simulink model "DisplayModel_Step4_start"  (R2013b)
settings: Solver=FixedStepDiscrete  StartTime=0.0  StopTime=10.0  FixedStep=0.2  RelTol=1e-3
settings Model: CovPath=LandingGearModes  CovMetricSettings=dcmw  CovHTMLOptions=-sRT=1 -aTS=1 -bRG=1 -bTC=1 -hTR=0 -nFC=0 -scm=1 -bcm=1 -xEv=0  CovModelRefEnable=off  Creator=siddhars  LastModifiedBy=rruff
settings OptimizationCC: InlineParams=on  ExpressionDepthLimit=2147483647  OptimizeModelRefInitCode=on  LifeSpan=1
settings DebuggingCC: StateNameClashWarn=warning
settings RTWCC: SystemTargetFile=ert.tlc  TemplateMakefile=ert_default_tmf  Description=Embedded Coder  ProcessScript=ert_make_rtw_hook  PortableWordSizes=on
settings CodeAppCC: IgnoreCustomStorageClasses=off  CustomSymbolStrType=$N$R$M  InternalIdentifier=Classic
settings ERTTargetCC: CodeReplacementLibrary=ANSI_C  GenerateSampleERTMain=on  InlinedParameterPlacement=NonHierarchical  ERTCustomFileTemplate=example_file_process.tlc
settings ConfigComp: Description=Design Verifier Custom Configuration Component  DVModelCoverageObjectives=MCDC  DVMaxTestCaseSteps=500  DVTestSuiteOptimization=CombinedObjectives (Nonlinear Extended)  DVSaveHarnessModel=on  DVModelReferenceHarness=on

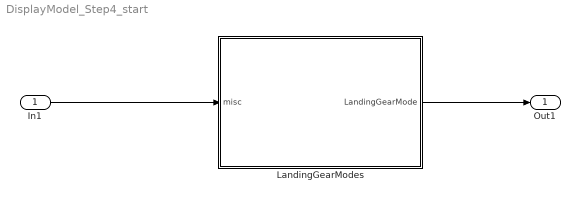
== system DisplayModel_Step4_start ==
  In1 : Inport  OutDataTypeStr=Bus: MiscData
  LandingGearModes : Stateflow chart  TreatAsAtomicUnit=on
  Out1 : Outport
  wires:
  LandingGearModes/1(LandingGearMode) -> Out1/1
  In1/1 -> LandingGearModes/1(misc)

== stateflow chart DisplayModel_Step4_start/LandingGearModes ==
  state LeftLock [parallel]
    settings: executionOrder=1
    state Unlocked
    state Locked
    (default) -> (junction 122)
    (junction 122) -> LeftLock.Unlocked [order 2]
    (junction 122) -> LeftLock.Locked [order 1] : [misc.LGLeftLock]
    LeftLock.Locked -> LeftLock.Unlocked : [~misc.LGLeftLock]
    LeftLock.Unlocked -> LeftLock.Locked : [misc.LGLeftLock]
  state RightLock [parallel]
    settings: executionOrder=2
    state Unlocked
    state Locked
    (default) -> (junction 136)
    (junction 136) -> RightLock.Unlocked [order 2]
    (junction 136) -> RightLock.Locked [order 1] : [misc.LGRightLock]
    RightLock.Locked -> RightLock.Unlocked : [~misc.LGRightLock]
    RightLock.Unlocked -> RightLock.Locked : [misc.LGRightLock]
  state WarningModes [parallel]
    settings: executionOrder=3
    state BothLocked
      entry:
      LandingGearMode = 1;
    state BothUnLocked
      entry:
      LandingGearMode = 3;
    state OnlyOneLocked
      entry:
      LandingGearMode = 2;
    (default) -> (junction 102)
    (junction 102) -> BothLocked [order 1] : [in(LeftLock.Locked) &&...
        | in(RightLock.Locked)]
    (junction 102) -> BothUnLocked [order 2] : [in(LeftLock.Unlocked) &&...
        | in(RightLock.Unlocked)]
    (junction 102) -> OnlyOneLocked [order 3]
    BothUnLocked -> OnlyOneLocked [order 2] : [in(LeftLock.Locked) ||...
        | in(RightLock.Locked)]
    OnlyOneLocked -> BothLocked [order 2] : [in(LeftLock.Locked) &&...
        | in(RightLock.Locked)]
    OnlyOneLocked -> BothUnLocked [order 1] : [in(LeftLock.Unlocked) &&...
        | in(RightLock.Unlocked)]
    BothLocked -> OnlyOneLocked [order 2] : [in(LeftLock.Unlocked) ||...
        | in(RightLock.Unlocked)]
    BothLocked -> BothUnLocked [order 1] : [in(LeftLock.Unlocked) &&...
        | in(RightLock.Unlocked)]
    BothUnLocked -> BothLocked [order 1] : [in(LeftLock.Locked) &&...
        | in(RightLock.Locked)]
  data: misc input Bus: MiscData; LandingGearMode output double size=1
